simulink model "TITAN_20160720_lec"  (R2016a)
settings: Solver=FixedStepDiscrete  SolverMode=SingleTasking  StartTime=0.0  StopTime=inf  FixedStep=SampleTime  RelTol=1e-3
values from neighbouring files (symbols this model uses):
  LegSampleTime = 0.30    (= 0.3)    [TitanAnalysis_20160720.m]
  SampleTime = 0.05    [TitanAnalysis_20160720.m]
  StepSize = SupportLegStep + IdlingLegStep    [TrajBreakup.m]
undefined symbols (not defined in the file or in its folder): LegTheta
libraries: arduinolib x52, simulink x26, dspswit3 x1
(part 1 of 2)
settings Model: SimulationMode=external  ExtModeTrigDuration=2  Creator=隆  LastModifiedBy=Deckadance
settings DataIOCC: LimitDataPoints=on  SaveFormat=Array
settings OptimizationCC: OptimizeModelRefInitCode=on  LifeSpan=Inf  MaxStackSize=64
settings DebuggingCC: UnderspecifiedInitializationDetection=Classic  MergeDetectMultiDrivingBlocksExec=none  AllowSymbolicDim=off
settings HardwareCC: ProdBitPerInt=16  ProdBitPerPointer=16  ProdLargestAtomicFloat=None  ProdWordSize=8  ProdHWDeviceType=Atmel->AVR  UseEmbeddedCoderFeatures=off  UseSimulinkCoderFeatures=off
settings ModelReferenceCC: PropagateSignalLabelsOutOfModel=off
settings RTWCC: SystemTargetFile=ert.tlc  HardwareBoard=Arduino Mega 2560  TemplateMakefile=ert_default_tmf  RTWVerbose=off  Toolchain=Arduino AVR v1.6.1  BuildConfiguration=Faster Runs
settings CodeAppCC: IgnoreCustomStorageClasses=off
settings ERTTargetCC: SupportContinuousTime=on  SupportNonInlinedSFcns=on  SupportVariableSizeSignals=on  ConvertIfToSwitch=off  SuppressUnreachableDefaultCases=off
settings ConfigComp: CovModelRefEnable=Off

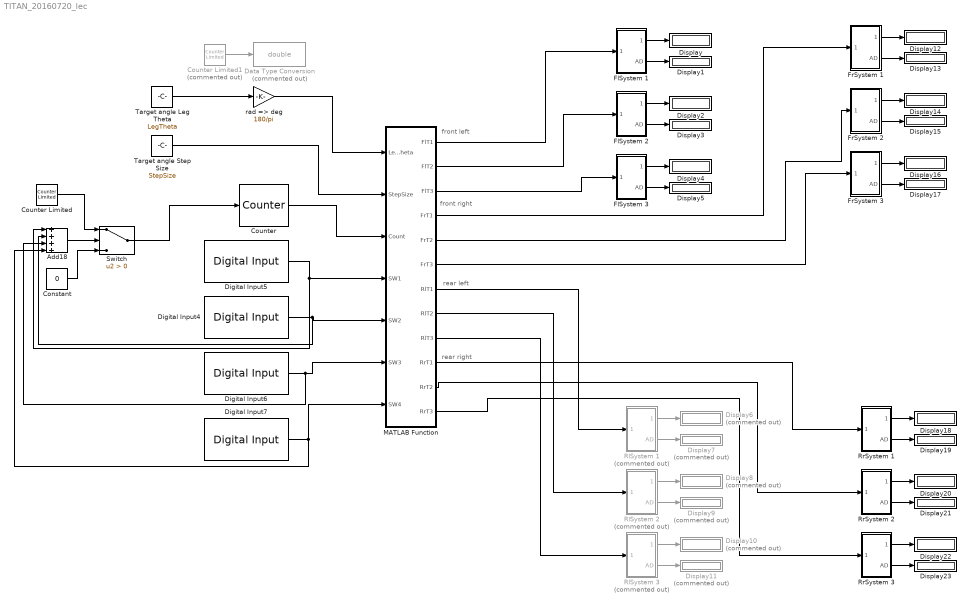
== system TITAN_20160720_lec ==
  note: rear right
  note: rear left
  note: front right
  note: front left
  Add18 : Sum  Inputs=++++
  Constant : Constant  Value=0
  Counter : dspswit3/Counter  Direction=Up  CountEvent=Either edge  CounterSize=User defined  MaxCount=StepSize-1  InitialCount=0  Output=Count  HitValue=32  ResetInput=off  SamplesPerFrame=1  Ts=1  CntDtype=double  HitDtype=Logical
  Counter Limited : simulink/Sources/Counter Limited  uplimit=1  tsamp=LegSampleTime
  Counter Limited1 : simulink/Sources/Counter Limited  Commented=on  uplimit=StepSize-1  tsamp=LegSampleTime
  Data Type Conversion : DataTypeConversion  Commented=on  OutDataTypeStr=double
  Digital Input4 : arduinolib/Digital Input  pinNumber=50  sampleTime=SampleTime  blockPlatform=arduino
  Digital Input5 : arduinolib/Digital Input  pinNumber=51  sampleTime=SampleTime  blockPlatform=arduino
  Digital Input6 : arduinolib/Digital Input  pinNumber=53  sampleTime=SampleTime  blockPlatform=arduino
  Digital Input7 : arduinolib/Digital Input  pinNumber=52  sampleTime=SampleTime  blockPlatform=arduino
  Display{,1..5,12..23} (18 alike) : Display
  Display{6..11} (6 alike) : Display  Commented=on
  FlSystem 1 : Subsystem
  FlSystem 2 : Subsystem
  FlSystem 3 : Subsystem
  FrSystem 1 : Subsystem
  FrSystem 2 : Subsystem
  FrSystem 3 : Subsystem
  MATLAB Function : MATLAB Function  TreatAsAtomicUnit=on
  RlSystem 1 : Subsystem  Commented=on
  RlSystem 2 : Subsystem  Commented=on
  RlSystem 3 : Subsystem  Commented=on
  RrSystem 1 : Subsystem
  RrSystem 2 : Subsystem
  RrSystem 3 : Subsystem
  Switch : Switch  Criteria=u2 > Threshold
  Target angle Leg Theta : Constant  Value=LegTheta  SampleTime=SampleTime
  Target angle Step Size : Constant  Value=StepSize  SampleTime=SampleTime
  rad => deg : Gain  Gain=180/pi
  wires:
  FlSystem 1/1(Angle) -> Display/1
  FlSystem 1/2(AD) -> Display1/1
  FlSystem 2/1(Angle) -> Display2/1
  FlSystem 2/2(AD) -> Display3/1
  FlSystem 3/1(Angle) -> Display4/1
  FlSystem 3/2(AD) -> Display5/1
  RlSystem 1/1(Angle) -> Display6/1
  RlSystem 1/2(AD) -> Display7/1
  RlSystem 2/1(Angle) -> Display8/1
  RlSystem 2/2(AD) -> Display9/1
  RlSystem 3/1(Angle) -> Display10/1
  RlSystem 3/2(AD) -> Display11/1
  FrSystem 1/1(Angle) -> Display12/1
  FrSystem 1/2(AD) -> Display13/1
  FrSystem 2/1(Angle) -> Display14/1
  FrSystem 2/2(AD) -> Display15/1
  FrSystem 3/1(Angle) -> Display16/1
  FrSystem 3/2(AD) -> Display17/1
  RrSystem 1/1(Angle) -> Display18/1
  RrSystem 1/2(AD) -> Display19/1
  RrSystem 2/1(Angle) -> Display20/1
  RrSystem 2/2(AD) -> Display21/1
  RrSystem 3/1(Angle) -> Display22/1
  RrSystem 3/2(AD) -> Display23/1
  MATLAB Function/4(FrT1) -> FrSystem 1/1(In1)
  Counter Limited1/1 -> Data Type Conversion/1
  Target angle Leg Theta/1 -> rad => deg/1
  MATLAB Function/5(FrT2) -> FrSystem 2/1(In1)
  MATLAB Function/6(FrT3) -> FrSystem 3/1(In1)
  MATLAB Function/3(FlT3) -> FlSystem 3/1(In1)
  MATLAB Function/2(FlT2) -> FlSystem 2/1(In1)
  MATLAB Function/1(FlT1) -> FlSystem 1/1(In1)
  MATLAB Function/7(RlT1) -> RlSystem 1/1(In1)
  MATLAB Function/8(RlT2) -> RlSystem 2/1(In1)
  MATLAB Function/9(RlT3) -> RlSystem 3/1(In1)
  MATLAB Function/10(RrT1) -> RrSystem 1/1(In1)
  MATLAB Function/11(RrT2) -> RrSystem 2/1(In1)
  MATLAB Function/12(RrT3) -> RrSystem 3/1(In1)
  Digital Input5/1 -> MATLAB Function/4(SW1), Add18/1
  Digital Input4/1 -> Add18/2, MATLAB Function/5(SW2)
  Counter/1 -> MATLAB Function/3(Count)
  rad => deg/1 -> MATLAB Function/1(LegTheta)
  Digital Input7/1 -> MATLAB Function/7(SW4), Add18/4
  Constant/1 -> Switch/3
  Add18/1 -> Switch/2
  Digital Input6/1 -> MATLAB Function/6(SW3), Add18/3
  Target angle Step Size/1 -> MATLAB Function/2(StepSize)
  Switch/1 -> Counter/1
  Counter Limited/1 -> Switch/1

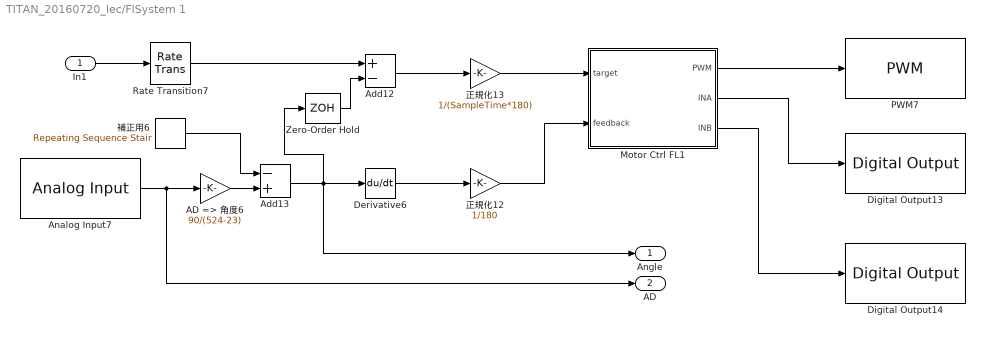
== system TITAN_20160720_lec/FlSystem 1 ==
  In1 : Inport
  AD => 角度6 : Gain  Gain=90/(524-23)
  Add12 : Sum  Inputs=+-
  Add13 : Sum  Inputs=-+
  Analog Input7 : arduinolib/Analog Input  pinNumber=0  sampleTime=SampleTime  blockPlatform=arduino
  Derivative6 : Derivative
  Digital Output13 : arduinolib/Digital Output  pinNumber=34  blockPlatform=arduino
  Digital Output14 : arduinolib/Digital Output  pinNumber=36  blockPlatform=arduino
  Motor Ctrl FL1 : Subsystem
  PWM7 : arduinolib/PWM  pinNumber=8  blockPlatform=arduino
  Rate Transition7 : RateTransition  OutPortSampleTime=SampleTime
  Zero-Order Hold : ZeroOrderHold  SampleTime=LegSampleTime
  正規化12 : Gain  Gain=1/180
  正規化13 : Gain  Gain=1/(SampleTime*180)
  補正用6 : simulink/Sources/Repeating Sequence Stair  OutValues=120.2  tsamp=SampleTime  OutMin=[]  OutMax=[]  OutDataTypeStr=double  OutputDataTypeScalingMode=double  OutDataType=fixdt(0,8)  ConRadixGroup=Best Precision: Vector-wise  OutScaling=2^-12
  Angle : Outport
  AD : Outport  Port=2
  wires:
  Derivative6/1 -> 正規化12/1
  Add13/1 -> Zero-Order Hold/1, Angle/1, Derivative6/1
  Motor Ctrl FL1/2(INA) -> Digital Output13/1
  Motor Ctrl FL1/3(INB) -> Digital Output14/1
  正規化12/1 -> Motor Ctrl FL1/2(feedback)
  Analog Input7/1 -> AD/1, AD => 角度6/1
  Motor Ctrl FL1/1(PWM) -> PWM7/1
  Rate Transition7/1 -> Add12/1
  正規化13/1 -> Motor Ctrl FL1/1(target)
  Add12/1 -> 正規化13/1
  AD => 角度6/1 -> Add13/2
  補正用6/1 -> Add13/1
  In1/1 -> Rate Transition7/1
  Zero-Order Hold/1 -> Add12/2

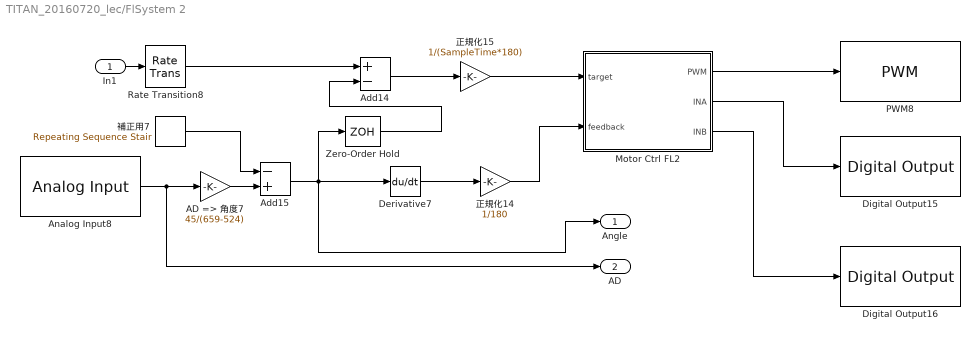
== system TITAN_20160720_lec/FlSystem 2 ==
  In1 : Inport
  AD => 角度7 : Gain  Gain=45/(659-524)
  Add14 : Sum  Inputs=+-
  Add15 : Sum  Inputs=-+
  Analog Input8 : arduinolib/Analog Input  pinNumber=1  sampleTime=SampleTime  blockPlatform=arduino
  Derivative7 : Derivative
  Digital Output15 : arduinolib/Digital Output  pinNumber=35  blockPlatform=arduino
  Digital Output16 : arduinolib/Digital Output  pinNumber=37  blockPlatform=arduino
  Motor Ctrl FL2 : Subsystem
  PWM8 : arduinolib/PWM  pinNumber=9  blockPlatform=arduino
  Rate Transition8 : RateTransition  OutPortSampleTime=SampleTime
  Zero-Order Hold : ZeroOrderHold  SampleTime=LegSampleTime
  正規化14 : Gain  Gain=1/180
  正規化15 : Gain  Gain=1/(SampleTime*180)
  補正用7 : simulink/Sources/Repeating Sequence Stair  OutValues=180  tsamp=SampleTime  OutMin=[]  OutMax=[]  OutDataTypeStr=double  OutputDataTypeScalingMode=double  OutDataType=fixdt(0,8)  ConRadixGroup=Best Precision: Vector-wise  OutScaling=2^-12
  Angle : Outport
  AD : Outport  Port=2
  wires:
  In1/1 -> Rate Transition8/1
  Derivative7/1 -> 正規化14/1
  Add15/1 -> Zero-Order Hold/1, Angle/1, Derivative7/1
  Motor Ctrl FL2/2(INA) -> Digital Output15/1
  Motor Ctrl FL2/3(INB) -> Digital Output16/1
  正規化14/1 -> Motor Ctrl FL2/2(feedback)
  Analog Input8/1 -> AD/1, AD => 角度7/1
  Motor Ctrl FL2/1(PWM) -> PWM8/1
  Rate Transition8/1 -> Add14/1
  正規化15/1 -> Motor Ctrl FL2/1(target)
  Add14/1 -> 正規化15/1
  AD => 角度7/1 -> Add15/2
  補正用7/1 -> Add15/1
  Zero-Order Hold/1 -> Add14/2

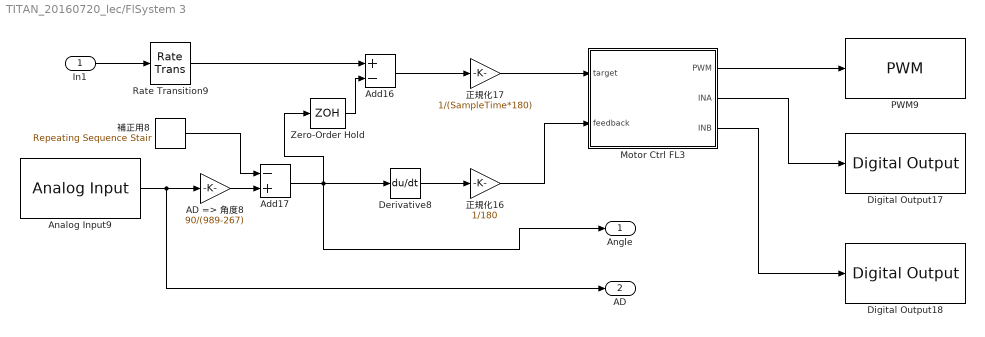
== system TITAN_20160720_lec/FlSystem 3 ==
  In1 : Inport
  AD => 角度8 : Gain  Gain=90/(989-267)
  Add16 : Sum  Inputs=+-
  Add17 : Sum  Inputs=-+
  Analog Input9 : arduinolib/Analog Input  pinNumber=2  sampleTime=SampleTime  blockPlatform=arduino
  Derivative8 : Derivative
  Digital Output17 : arduinolib/Digital Output  pinNumber=41  blockPlatform=arduino
  Digital Output18 : arduinolib/Digital Output  pinNumber=39  blockPlatform=arduino
  Motor Ctrl FL3 : Subsystem
  PWM9 : arduinolib/PWM  pinNumber=11  blockPlatform=arduino
  Rate Transition9 : RateTransition  OutPortSampleTime=SampleTime
  Zero-Order Hold : ZeroOrderHold  SampleTime=LegSampleTime
  正規化16 : Gain  Gain=1/180
  正規化17 : Gain  Gain=1/(SampleTime*180)
  補正用8 : simulink/Sources/Repeating Sequence Stair  OutValues=33.28+90  tsamp=SampleTime  OutMin=[]  OutMax=[]  OutDataTypeStr=double  OutputDataTypeScalingMode=double  OutDataType=fixdt(0,8)  ConRadixGroup=Best Precision: Vector-wise  OutScaling=2^-12
  Angle : Outport
  AD : Outport  Port=2
  wires:
  Derivative8/1 -> 正規化16/1
  Add17/1 -> Zero-Order Hold/1, Angle/1, Derivative8/1
  Motor Ctrl FL3/2(INA) -> Digital Output17/1
  Motor Ctrl FL3/3(INB) -> Digital Output18/1
  正規化16/1 -> Motor Ctrl FL3/2(feedback)
  Analog Input9/1 -> AD/1, AD => 角度8/1
  Motor Ctrl FL3/1(PWM) -> PWM9/1
  Rate Transition9/1 -> Add16/1
  正規化17/1 -> Motor Ctrl FL3/1(target)
  Add16/1 -> 正規化17/1
  AD => 角度8/1 -> Add17/2
  補正用8/1 -> Add17/1
  In1/1 -> Rate Transition9/1
  Zero-Order Hold/1 -> Add16/2

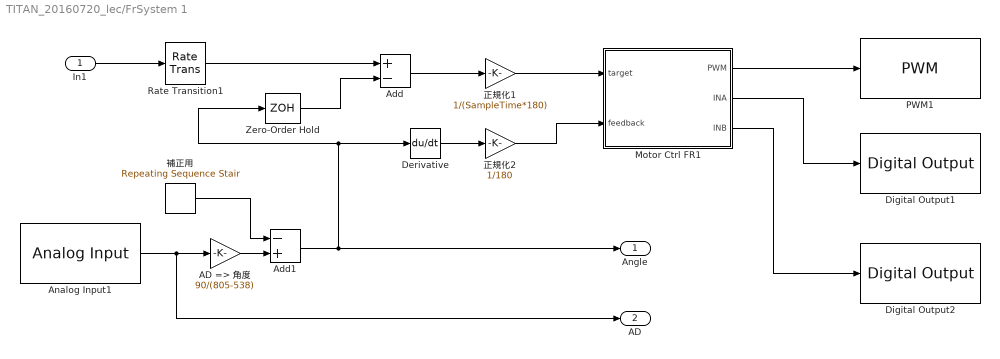
== system TITAN_20160720_lec/FrSystem 1 ==
  In1 : Inport
  AD => 角度 : Gain  Gain=90/(805-538)
  Add : Sum  Inputs=+-
  Add1 : Sum  Inputs=-+
  Analog Input1 : arduinolib/Analog Input  pinNumber=3  sampleTime=SampleTime  blockPlatform=arduino
  Derivative : Derivative
  Digital Output1 : arduinolib/Digital Output  pinNumber=42  blockPlatform=arduino
  Digital Output2 : arduinolib/Digital Output  pinNumber=44  blockPlatform=arduino
  Motor Ctrl FR1 : Subsystem
  PWM1 : arduinolib/PWM  pinNumber=12  blockPlatform=arduino
  Rate Transition1 : RateTransition  OutPortSampleTime=SampleTime
  Zero-Order Hold : ZeroOrderHold  SampleTime=LegSampleTime
  正規化1 : Gain  Gain=1/(SampleTime*180)
  正規化2 : Gain  Gain=1/180
  補正用 : simulink/Sources/Repeating Sequence Stair  OutValues=180  tsamp=SampleTime  OutMin=[]  OutMax=[]  OutDataTypeStr=double  OutputDataTypeScalingMode=double  OutDataType=fixdt(0,8)  ConRadixGroup=Best Precision: Vector-wise  OutScaling=2^-12
  Angle : Outport
  AD : Outport  Port=2
  wires:
  In1/1 -> Rate Transition1/1
  Motor Ctrl FR1/2(INA) -> Digital Output1/1
  Motor Ctrl FR1/3(INB) -> Digital Output2/1
  Derivative/1 -> 正規化2/1
  Analog Input1/1 -> AD/1, AD => 角度/1
  Motor Ctrl FR1/1(PWM) -> PWM1/1
  Rate Transition1/1 -> Add/1
  AD => 角度/1 -> Add1/2
  Add/1 -> 正規化1/1
  補正用/1 -> Add1/1
  正規化1/1 -> Motor Ctrl FR1/1(target)
  正規化2/1 -> Motor Ctrl FR1/2(feedback)
  Add1/1 -> Derivative/1, Zero-Order Hold/1, Angle/1
  Zero-Order Hold/1 -> Add/2

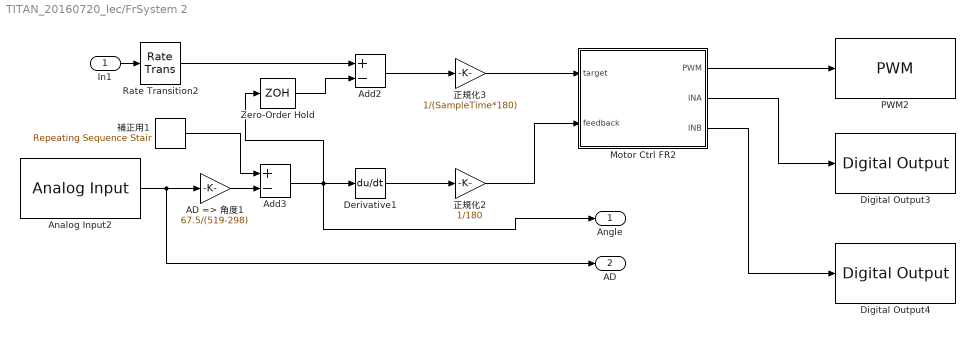
== system TITAN_20160720_lec/FrSystem 2 ==
  In1 : Inport
  AD => 角度1 : Gain  Gain=67.5/(519-298)
  Add2 : Sum  Inputs=+-
  Add3 : Sum  Inputs=+-
  Analog Input2 : arduinolib/Analog Input  pinNumber=4  sampleTime=SampleTime  blockPlatform=arduino
  Derivative1 : Derivative
  Digital Output3 : arduinolib/Digital Output  pinNumber=45  blockPlatform=arduino
  Digital Output4 : arduinolib/Digital Output  pinNumber=43  blockPlatform=arduino
  Motor Ctrl FR2 : Subsystem
  PWM2 : arduinolib/PWM  pinNumber=13  blockPlatform=arduino
  Rate Transition2 : RateTransition  OutPortSampleTime=SampleTime
  Zero-Order Hold : ZeroOrderHold  SampleTime=LegSampleTime
  正規化2 : Gain  Gain=1/180
  正規化3 : Gain  Gain=1/(SampleTime*180)
  補正用1 : simulink/Sources/Repeating Sequence Stair  OutValues=158.5  tsamp=SampleTime  OutMin=[]  OutMax=[]  OutDataTypeStr=double  OutputDataTypeScalingMode=double  OutDataType=fixdt(0,8)  ConRadixGroup=Best Precision: Vector-wise  OutScaling=2^-12
  Angle : Outport
  AD : Outport  Port=2
  wires:
  In1/1 -> Rate Transition2/1
  Derivative1/1 -> 正規化2/1
  Add3/1 -> Angle/1, Zero-Order Hold/1, Derivative1/1
  Motor Ctrl FR2/2(INA) -> Digital Output3/1
  Motor Ctrl FR2/3(INB) -> Digital Output4/1
  正規化2/1 -> Motor Ctrl FR2/2(feedback)
  Analog Input2/1 -> AD/1, AD => 角度1/1
  Motor Ctrl FR2/1(PWM) -> PWM2/1
  正規化3/1 -> Motor Ctrl FR2/1(target)
  Rate Transition2/1 -> Add2/1
  Add2/1 -> 正規化3/1
  AD => 角度1/1 -> Add3/2
  補正用1/1 -> Add3/1
  Zero-Order Hold/1 -> Add2/2

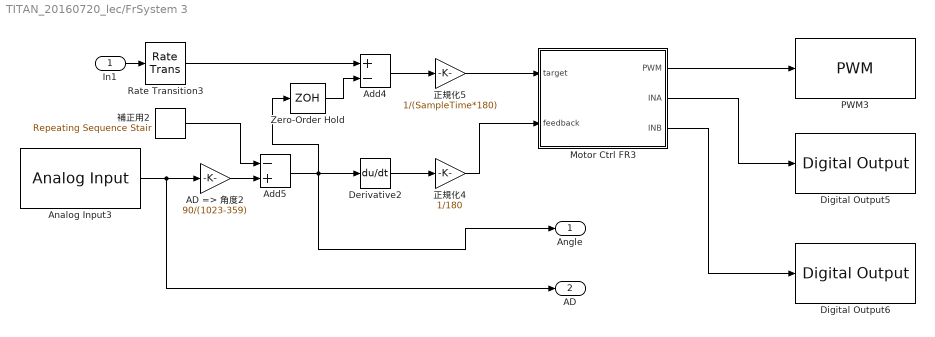
== system TITAN_20160720_lec/FrSystem 3 ==
  In1 : Inport
  AD => 角度2 : Gain  Gain=90/(1023-359)
  Add4 : Sum  Inputs=+-
  Add5 : Sum  Inputs=-+
  Analog Input3 : arduinolib/Analog Input  pinNumber=5  sampleTime=SampleTime  blockPlatform=arduino
  Derivative2 : Derivative
  Digital Output5 : arduinolib/Digital Output  pinNumber=38  blockPlatform=arduino
  Digital Output6 : arduinolib/Digital Output  pinNumber=40  blockPlatform=arduino
  Motor Ctrl FR3 : Subsystem
  PWM3 : arduinolib/PWM  pinNumber=10  blockPlatform=arduino
  Rate Transition3 : RateTransition  OutPortSampleTime=SampleTime
  Zero-Order Hold : ZeroOrderHold  SampleTime=LegSampleTime
  正規化4 : Gain  Gain=1/180
  正規化5 : Gain  Gain=1/(SampleTime*180)
  補正用2 : simulink/Sources/Repeating Sequence Stair  OutValues=47.3+90  tsamp=SampleTime  OutMin=[]  OutMax=[]  OutDataTypeStr=double  OutputDataTypeScalingMode=double  OutDataType=fixdt(0,8)  ConRadixGroup=Best Precision: Vector-wise  OutScaling=2^-12
  Angle : Outport
  AD : Outport  Port=2
  wires:
  In1/1 -> Rate Transition3/1
  Derivative2/1 -> 正規化4/1
  Add5/1 -> Zero-Order Hold/1, Angle/1, Derivative2/1
  Motor Ctrl FR3/2(INA) -> Digital Output5/1
  Motor Ctrl FR3/3(INB) -> Digital Output6/1
  正規化4/1 -> Motor Ctrl FR3/2(feedback)
  Analog Input3/1 -> AD/1, AD => 角度2/1
  Motor Ctrl FR3/1(PWM) -> PWM3/1
  Rate Transition3/1 -> Add4/1
  Add4/1 -> 正規化5/1
  AD => 角度2/1 -> Add5/2
  補正用2/1 -> Add5/1
  正規化5/1 -> Motor Ctrl FR3/1(target)
  Zero-Order Hold/1 -> Add4/2

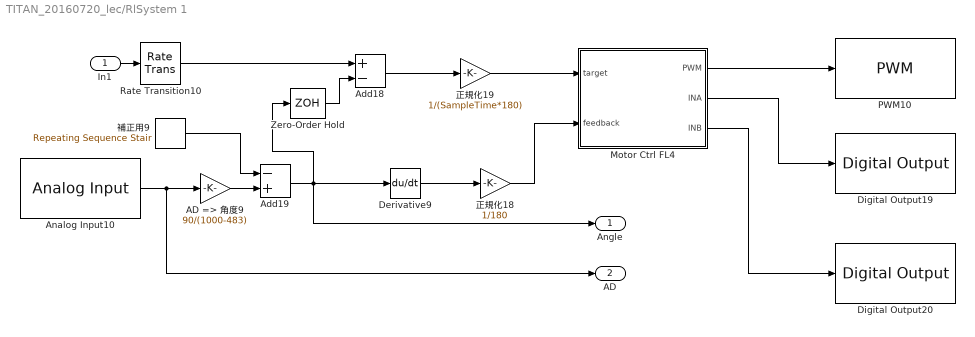
== system TITAN_20160720_lec/RlSystem 1 ==
  In1 : Inport
  AD => 角度9 : Gain  Gain=90/(1000-483)
  Add18 : Sum  Inputs=+-
  Add19 : Sum  Inputs=-+
  Analog Input10 : arduinolib/Analog Input  pinNumber=9  sampleTime=SampleTime  blockPlatform=arduino
  Derivative9 : Derivative
  Digital Output19 : arduinolib/Digital Output  pinNumber=30  blockPlatform=arduino
  Digital Output20 : arduinolib/Digital Output  pinNumber=32  blockPlatform=arduino
  Motor Ctrl FL4 : Subsystem
  PWM10 : arduinolib/PWM  pinNumber=6  blockPlatform=arduino
  Rate Transition10 : RateTransition  OutPortSampleTime=SampleTime
  Zero-Order Hold : ZeroOrderHold  SampleTime=LegSampleTime
  正規化18 : Gain  Gain=1/180
  正規化19 : Gain  Gain=1/(SampleTime*180)
  補正用9 : simulink/Sources/Repeating Sequence Stair  OutValues=83.38  tsamp=SampleTime  OutMin=[]  OutMax=[]  OutDataTypeStr=double  OutputDataTypeScalingMode=double  OutDataType=fixdt(0,8)  ConRadixGroup=Best Precision: Vector-wise  OutScaling=2^-12
  Angle : Outport
  AD : Outport  Port=2
  wires:
  In1/1 -> Rate Transition10/1
  Derivative9/1 -> 正規化18/1
  Add19/1 -> Zero-Order Hold/1, Angle/1, Derivative9/1
  Motor Ctrl FL4/2(INA) -> Digital Output19/1
  Motor Ctrl FL4/3(INB) -> Digital Output20/1
  正規化18/1 -> Motor Ctrl FL4/2(feedback)
  Analog Input10/1 -> AD/1, AD => 角度9/1
  Motor Ctrl FL4/1(PWM) -> PWM10/1
  Rate Transition10/1 -> Add18/1
  正規化19/1 -> Motor Ctrl FL4/1(target)
  Add18/1 -> 正規化19/1
  AD => 角度9/1 -> Add19/2
  補正用9/1 -> Add19/1
  Zero-Order Hold/1 -> Add18/2

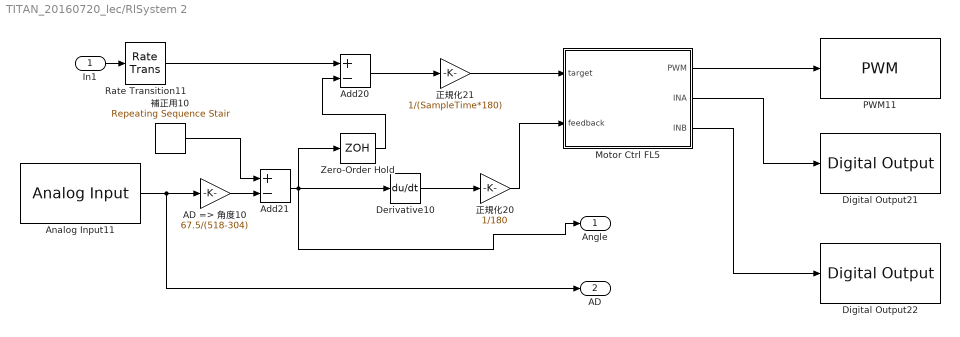
== system TITAN_20160720_lec/RlSystem 2 ==
  In1 : Inport
  AD => 角度10 : Gain  Gain=67.5/(518-304)
  Add20 : Sum  Inputs=+-
  Add21 : Sum  Inputs=+-
  Analog Input11 : arduinolib/Analog Input  pinNumber=10  sampleTime=SampleTime  blockPlatform=arduino
  Derivative10 : Derivative
  Digital Output21 : arduinolib/Digital Output  pinNumber=33  blockPlatform=arduino
  Digital Output22 : arduinolib/Digital Output  pinNumber=31  blockPlatform=arduino
  Motor Ctrl FL5 : Subsystem
  PWM11 : arduinolib/PWM  pinNumber=7  blockPlatform=arduino
  Rate Transition11 : RateTransition  OutPortSampleTime=SampleTime
  Zero-Order Hold : ZeroOrderHold  SampleTime=LegSampleTime
  正規化20 : Gain  Gain=1/180
  正規化21 : Gain  Gain=1/(SampleTime*180)
  補正用10 : simulink/Sources/Repeating Sequence Stair  OutValues=161.5  tsamp=SampleTime  OutMin=[]  OutMax=[]  OutDataTypeStr=double  OutputDataTypeScalingMode=double  OutDataType=fixdt(0,8)  ConRadixGroup=Best Precision: Vector-wise  OutScaling=2^-12
  Angle : Outport
  AD : Outport  Port=2
  wires:
  In1/1 -> Rate Transition11/1
  Derivative10/1 -> 正規化20/1
  Add21/1 -> Zero-Order Hold/1, Angle/1, Derivative10/1
  Motor Ctrl FL5/2(INA) -> Digital Output21/1
  Motor Ctrl FL5/3(INB) -> Digital Output22/1
  正規化20/1 -> Motor Ctrl FL5/2(feedback)
  Analog Input11/1 -> AD/1, AD => 角度10/1
  Motor Ctrl FL5/1(PWM) -> PWM11/1
  Rate Transition11/1 -> Add20/1
  正規化21/1 -> Motor Ctrl FL5/1(target)
  Add20/1 -> 正規化21/1
  AD => 角度10/1 -> Add21/2
  補正用10/1 -> Add21/1
  Zero-Order Hold/1 -> Add20/2

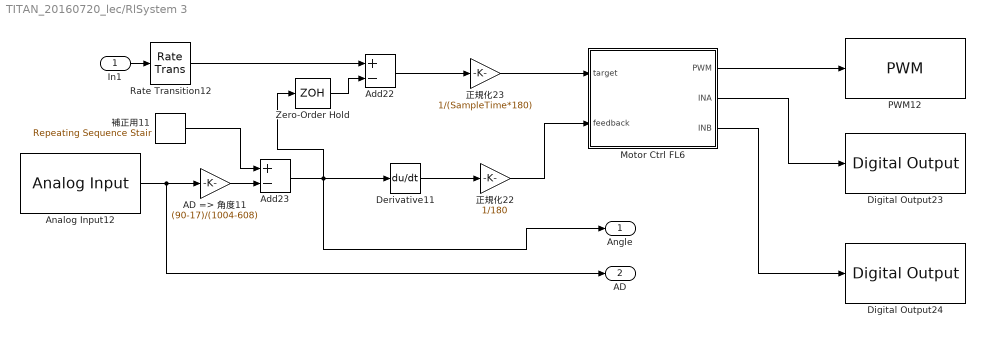
== system TITAN_20160720_lec/RlSystem 3 ==
  In1 : Inport
  AD => 角度11 : Gain  Gain=(90-17)/(1004-608)
  Add22 : Sum  Inputs=+-
  Add23 : Sum  Inputs=+-
  Analog Input12 : arduinolib/Analog Input  pinNumber=11  sampleTime=SampleTime  blockPlatform=arduino
  Derivative11 : Derivative
  Digital Output23 : arduinolib/Digital Output  pinNumber=26  blockPlatform=arduino
  Digital Output24 : arduinolib/Digital Output  pinNumber=28  blockPlatform=arduino
  Motor Ctrl FL6 : Subsystem
  PWM12 : arduinolib/PWM  pinNumber=4  blockPlatform=arduino
  Rate Transition12 : RateTransition  OutPortSampleTime=SampleTime
  Zero-Order Hold : ZeroOrderHold  SampleTime=LegSampleTime
  正規化22 : Gain  Gain=1/180
  正規化23 : Gain  Gain=1/(SampleTime*180)
  補正用11 : simulink/Sources/Repeating Sequence Stair  OutValues=110-90  tsamp=SampleTime  OutMin=[]  OutMax=[]  OutDataTypeStr=double  OutputDataTypeScalingMode=double  OutDataType=fixdt(0,8)  ConRadixGroup=Best Precision: Vector-wise  OutScaling=2^-12
  Angle : Outport
  AD : Outport  Port=2
  wires:
  Derivative11/1 -> 正規化22/1
  Motor Ctrl FL6/2(INA) -> Digital Output23/1
  Motor Ctrl FL6/3(INB) -> Digital Output24/1
  正規化22/1 -> Motor Ctrl FL6/2(feedback)
  Analog Input12/1 -> AD/1, AD => 角度11/1
  Motor Ctrl FL6/1(PWM) -> PWM12/1
  Rate Transition12/1 -> Add22/1
  正規化23/1 -> Motor Ctrl FL6/1(target)
  Add22/1 -> 正規化23/1
  AD => 角度11/1 -> Add23/2
  補正用11/1 -> Add23/1
  In1/1 -> Rate Transition12/1
  Zero-Order Hold/1 -> Add22/2
  Add23/1 -> Zero-Order Hold/1, Angle/1, Derivative11/1

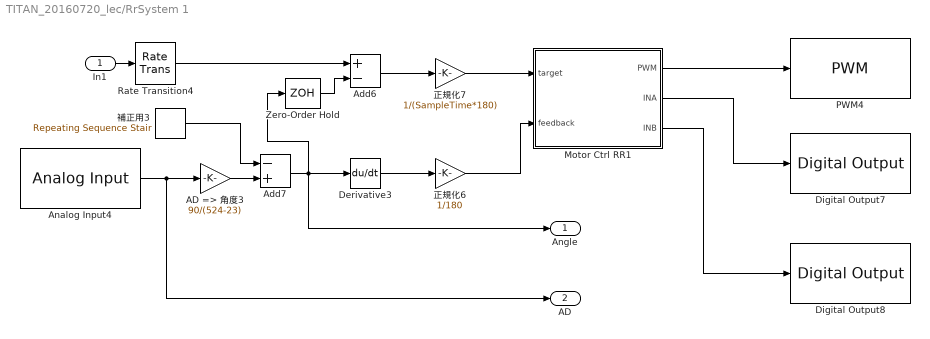
== system TITAN_20160720_lec/RrSystem 1 ==
  In1 : Inport
  AD => 角度3 : Gain  Gain=90/(524-23)
  Add6 : Sum  Inputs=+-
  Add7 : Sum  Inputs=-+
  Analog Input4 : arduinolib/Analog Input  pinNumber=6  sampleTime=SampleTime  blockPlatform=arduino
  Derivative3 : Derivative
  Digital Output7 : arduinolib/Digital Output  pinNumber=22  blockPlatform=arduino
  Digital Output8 : arduinolib/Digital Output  pinNumber=24  blockPlatform=arduino
  Motor Ctrl RR1 : Subsystem
  PWM4 : arduinolib/PWM  pinNumber=2  blockPlatform=arduino
  Rate Transition4 : RateTransition  OutPortSampleTime=SampleTime
  Zero-Order Hold : ZeroOrderHold  SampleTime=LegSampleTime
  正規化6 : Gain  Gain=1/180
  正規化7 : Gain  Gain=1/(SampleTime*180)
  補正用3 : simulink/Sources/Repeating Sequence Stair  OutValues=93.77  tsamp=SampleTime  OutMin=[]  OutMax=[]  OutDataTypeStr=double  OutputDataTypeScalingMode=double  OutDataType=fixdt(0,8)  ConRadixGroup=Best Precision: Vector-wise  OutScaling=2^-12
  Angle : Outport
  AD : Outport  Port=2
  wires:
  In1/1 -> Rate Transition4/1
  Derivative3/1 -> 正規化6/1
  Add7/1 -> Zero-Order Hold/1, Angle/1, Derivative3/1
  Motor Ctrl RR1/2(INA) -> Digital Output7/1
  Motor Ctrl RR1/3(INB) -> Digital Output8/1
  正規化6/1 -> Motor Ctrl RR1/2(feedback)
  Analog Input4/1 -> AD/1, AD => 角度3/1
  Motor Ctrl RR1/1(PWM) -> PWM4/1
  Rate Transition4/1 -> Add6/1
  Add6/1 -> 正規化7/1
  正規化7/1 -> Motor Ctrl RR1/1(target)
  補正用3/1 -> Add7/1
  AD => 角度3/1 -> Add7/2
  Zero-Order Hold/1 -> Add6/2

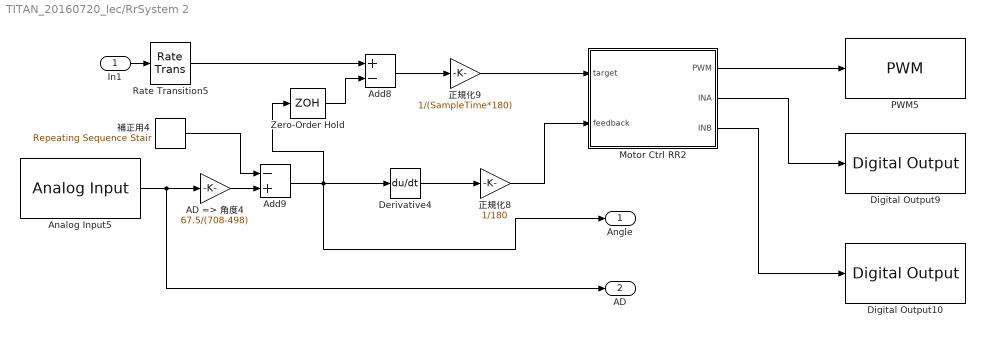
== system TITAN_20160720_lec/RrSystem 2 ==
  In1 : Inport
  AD => 角度4 : Gain  Gain=67.5/(708-498)
  Add8 : Sum  Inputs=+-
  Add9 : Sum  Inputs=-+
  Analog Input5 : arduinolib/Analog Input  pinNumber=7  sampleTime=SampleTime  blockPlatform=arduino
  Derivative4 : Derivative
  Digital Output10 : arduinolib/Digital Output  pinNumber=25  blockPlatform=arduino
  Digital Output9 : arduinolib/Digital Output  pinNumber=23  blockPlatform=arduino
  Motor Ctrl RR2 : Subsystem
  PWM5 : arduinolib/PWM  pinNumber=3  blockPlatform=arduino
  Rate Transition5 : RateTransition  OutPortSampleTime=SampleTime
  Zero-Order Hold : ZeroOrderHold  SampleTime=LegSampleTime
  正規化8 : Gain  Gain=1/180
  正規化9 : Gain  Gain=1/(SampleTime*180)
  補正用4 : simulink/Sources/Repeating Sequence Stair  OutValues=160.7  tsamp=SampleTime  OutMin=[]  OutMax=[]  OutDataTypeStr=double  OutputDataTypeScalingMode=double  OutDataType=fixdt(0,8)  ConRadixGroup=Best Precision: Vector-wise  OutScaling=2^-12
  Angle : Outport
  AD : Outport  Port=2
  wires:
  In1/1 -> Rate Transition5/1
  Derivative4/1 -> 正規化8/1
  Add9/1 -> Zero-Order Hold/1, Angle/1, Derivative4/1
  Motor Ctrl RR2/2(INA) -> Digital Output9/1
  Motor Ctrl RR2/3(INB) -> Digital Output10/1
  正規化8/1 -> Motor Ctrl RR2/2(feedback)
  Analog Input5/1 -> AD/1, AD => 角度4/1
  Motor Ctrl RR2/1(PWM) -> PWM5/1
  Rate Transition5/1 -> Add8/1
  正規化9/1 -> Motor Ctrl RR2/1(target)
  Add8/1 -> 正規化9/1
  AD => 角度4/1 -> Add9/2
  補正用4/1 -> Add9/1
  Zero-Order Hold/1 -> Add8/2

== system TITAN_20160720_lec/RrSystem 3 ==
  In1 : Inport
  AD => 角度5 : Gain  Gain=(134-17)/(1003-21)
  Add10 : Sum  Inputs=+-
  Add11 : Sum  Inputs=+-
  Analog Input6 : arduinolib/Analog Input  pinNumber=8  sampleTime=SampleTime  blockPlatform=arduino
  Derivative5 : Derivative
  Digital Output11 : arduinolib/Digital Output  pinNumber=29  blockPlatform=arduino
  Digital Output12 : arduinolib/Digital Output  pinNumber=27  blockPlatform=arduino
  Motor Ctrl RR3 : Subsystem
  PWM6 : arduinolib/PWM  pinNumber=5  blockPlatform=arduino
  Rate Transition6 : RateTransition  OutPortSampleTime=SampleTime
  Zero-Order Hold : ZeroOrderHold  SampleTime=LegSampleTime
  正規化10 : Gain  Gain=1/180
  正規化11 : Gain  Gain=1/(SampleTime*180)
  補正用5 : simulink/Sources/Repeating Sequence Stair  OutValues=78.06-90  tsamp=SampleTime  OutMin=[]  OutMax=[]  OutDataTypeStr=double  OutputDataTypeScalingMode=double  OutDataType=fixdt(0,8)  ConRadixGroup=Best Precision: Vector-wise  OutScaling=2^-12
  Angle : Outport
  AD : Outport  Port=2
  wires:
  In1/1 -> Rate Transition6/1
  Derivative5/1 -> 正規化10/1
  Add11/1 -> Zero-Order Hold/1, Angle/1, Derivative5/1
  Motor Ctrl RR3/2(INA) -> Digital Output11/1
  Motor Ctrl RR3/3(INB) -> Digital Output12/1
  正規化10/1 -> Motor Ctrl RR3/2(feedback)
  Analog Input6/1 -> AD/1, AD => 角度5/1
  Motor Ctrl RR3/1(PWM) -> PWM6/1
  Rate Transition6/1 -> Add10/1
  Add10/1 -> 正規化11/1
  正規化11/1 -> Motor Ctrl RR3/1(target)
  補正用5/1 -> Add11/1
  AD => 角度5/1 -> Add11/2
  Zero-Order Hold/1 -> Add10/2

== system TITAN_20160720_lec/FlSystem 1/Motor Ctrl FL1 ==
  note: motor driver
  target : Inport
  feedback : Inport  Port=2
  Abs : Abs
  Add : Sum  Inputs=+-
  Discrete PID Controller : simulink/Continuous/PID Controller  Controller=PID  TimeDomain=Discrete-time  SampleTime=SampleTime  IntegratorMethod=Trapezoidal  FilterMethod=Forward Euler  Form=Parallel  UseFilter=on  ControllerParametersSource=internal  P=0.25  I=0  D=0  N=100  InitialConditionSource=internal  InitialConditionForIntegrator=0  InitialConditionForFilter=0  ExternalReset=none  LimitOutput=on  UpperSaturationLimit=1  LowerSaturationLimit=-1  LinearizeAsGain=off  AntiWindupMode=none  Kb=1  TrackingMode=off  Kt=1  PParamMin=[]  PParamMax=[]  IParamMin=[]  IParamMax=[]  DParamMin=[]  DParamMax=[]  NParamMin=[]  NParamMax=[]  KbParamMin=[]  KbParamMax=[]  KtParamMin=[]  KtParamMax=[]  POutMin=[]  POutMax=[]  IOutMin=[]  IOutMax=[]  DOutMin=[]  DOutMax=[]  NOutMin=[]  NOutMax=[]  KbOutMin=[]  KbOutMax=[]  KtOutMin=[]  KtOutMax=[]  IntegratorOutMin=[]  IntegratorOutMax=[]  FilterOutMin=[]  FilterOutMax=[]  SumOutMin=[]  SumOutMax=[]  SumI1OutMin=[]  SumI1OutMax=[]  SumI2OutMin=[]  SumI2OutMax=[]  SumI3OutMin=[]  SumI3OutMax=[]  SumDOutMin=[]  SumDOutMax=[]  SaturationOutMin=[]  SaturationOutMax=[]  IntegratorContinuousStateAttributes=''  IntegratorStateMustResolveToSignalObject=off  IntegratorRTWStateStorageClass=Auto  FilterContinuousStateAttributes=''  FilterStateMustResolveToSignalObject=off  FilterRTWStateStorageClass=Auto  DifferentiatorICPrevScaledInput=0  DifferentiatorOutMin=[]  DifferentiatorOutMax=[]
  Gain : Gain  Gain=255
  Saturation : Saturate  UpperLimit=1  LowerLimit=0
  Saturation1 : Saturate  UpperLimit=1  LowerLimit=0
  Saturation2 : Saturate  UpperLimit=1  LowerLimit=0
  Sign : Signum
  Unary Minus : UnaryMinus
  PWM : Outport
  INA : Outport  Port=2
  INB : Outport  Port=3
  wires:
  feedback/1 -> Add/2
  Abs/1 -> Saturation2/1
  Sign/1 -> Unary Minus/1, Saturation/1
  Discrete PID Controller/1 -> Abs/1, Sign/1
  Saturation/1 -> INA/1
  Saturation1/1 -> INB/1
  Unary Minus/1 -> Saturation1/1
  target/1 -> Add/1
  Saturation2/1 -> Gain/1
  Gain/1 -> PWM/1
  Add/1 -> Discrete PID Controller/1

== system TITAN_20160720_lec/FlSystem 2/Motor Ctrl FL2 ==
  target : Inport
  feedback : Inport  Port=2
  Abs : Abs
  Add : Sum  Inputs=+-
  Discrete PID Controller : simulink/Continuous/PID Controller  Controller=PID  TimeDomain=Discrete-time  SampleTime=SampleTime  IntegratorMethod=Trapezoidal  FilterMethod=Forward Euler  Form=Parallel  UseFilter=on  ControllerParametersSource=internal  P=0.2  I=0  D=0  N=100  InitialConditionSource=internal  InitialConditionForIntegrator=0  InitialConditionForFilter=0  ExternalReset=none  LimitOutput=on  UpperSaturationLimit=1  LowerSaturationLimit=-1  LinearizeAsGain=off  AntiWindupMode=none  Kb=1  TrackingMode=off  Kt=1  PParamMin=[]  PParamMax=[]  IParamMin=[]  IParamMax=[]  DParamMin=[]  DParamMax=[]  NParamMin=[]  NParamMax=[]  KbParamMin=[]  KbParamMax=[]  KtParamMin=[]  KtParamMax=[]  POutMin=[]  POutMax=[]  IOutMin=[]  IOutMax=[]  DOutMin=[]  DOutMax=[]  NOutMin=[]  NOutMax=[]  KbOutMin=[]  KbOutMax=[]  KtOutMin=[]  KtOutMax=[]  IntegratorOutMin=[]  IntegratorOutMax=[]  FilterOutMin=[]  FilterOutMax=[]  SumOutMin=[]  SumOutMax=[]  SumI1OutMin=[]  SumI1OutMax=[]  SumI2OutMin=[]  SumI2OutMax=[]  SumI3OutMin=[]  SumI3OutMax=[]  SumDOutMin=[]  SumDOutMax=[]  SaturationOutMin=[]  SaturationOutMax=[]  IntegratorContinuousStateAttributes=''  IntegratorStateMustResolveToSignalObject=off  IntegratorRTWStateStorageClass=Auto  FilterContinuousStateAttributes=''  FilterStateMustResolveToSignalObject=off  FilterRTWStateStorageClass=Auto  DifferentiatorICPrevScaledInput=0  DifferentiatorOutMin=[]  DifferentiatorOutMax=[]
  Gain : Gain  Gain=255
  Saturation : Saturate  UpperLimit=1  LowerLimit=0
  Saturation1 : Saturate  UpperLimit=1  LowerLimit=0
  Saturation2 : Saturate  UpperLimit=1  LowerLimit=0
  Sign : Signum
  Unary Minus : UnaryMinus
  PWM : Outport
  INA : Outport  Port=2
  INB : Outport  Port=3
  wires:
  feedback/1 -> Add/2
  Abs/1 -> Saturation2/1
  Sign/1 -> Unary Minus/1, Saturation/1
  Discrete PID Controller/1 -> Abs/1, Sign/1
  Saturation/1 -> INA/1
  Saturation1/1 -> INB/1
  Unary Minus/1 -> Saturation1/1
  target/1 -> Add/1
  Saturation2/1 -> Gain/1
  Gain/1 -> PWM/1
  Add/1 -> Discrete PID Controller/1

== system TITAN_20160720_lec/FlSystem 3/Motor Ctrl FL3 ==
  target : Inport
  feedback : Inport  Port=2
  Abs : Abs
  Add : Sum  Inputs=+-
  Discrete PID Controller : simulink/Continuous/PID Controller  Controller=PID  TimeDomain=Discrete-time  SampleTime=SampleTime  IntegratorMethod=Trapezoidal  FilterMethod=Forward Euler  Form=Parallel  UseFilter=on  ControllerParametersSource=internal  P=0.2  I=0  D=0  N=100  InitialConditionSource=internal  InitialConditionForIntegrator=0  InitialConditionForFilter=0  ExternalReset=none  LimitOutput=on  UpperSaturationLimit=1  LowerSaturationLimit=-1  LinearizeAsGain=off  AntiWindupMode=none  Kb=1  TrackingMode=off  Kt=1  PParamMin=[]  PParamMax=[]  IParamMin=[]  IParamMax=[]  DParamMin=[]  DParamMax=[]  NParamMin=[]  NParamMax=[]  KbParamMin=[]  KbParamMax=[]  KtParamMin=[]  KtParamMax=[]  POutMin=[]  POutMax=[]  IOutMin=[]  IOutMax=[]  DOutMin=[]  DOutMax=[]  NOutMin=[]  NOutMax=[]  KbOutMin=[]  KbOutMax=[]  KtOutMin=[]  KtOutMax=[]  IntegratorOutMin=[]  IntegratorOutMax=[]  FilterOutMin=[]  FilterOutMax=[]  SumOutMin=[]  SumOutMax=[]  SumI1OutMin=[]  SumI1OutMax=[]  SumI2OutMin=[]  SumI2OutMax=[]  SumI3OutMin=[]  SumI3OutMax=[]  SumDOutMin=[]  SumDOutMax=[]  SaturationOutMin=[]  SaturationOutMax=[]  IntegratorContinuousStateAttributes=''  IntegratorStateMustResolveToSignalObject=off  IntegratorRTWStateStorageClass=Auto  FilterContinuousStateAttributes=''  FilterStateMustResolveToSignalObject=off  FilterRTWStateStorageClass=Auto  DifferentiatorICPrevScaledInput=0  DifferentiatorOutMin=[]  DifferentiatorOutMax=[]
  Gain : Gain  Gain=255
  Saturation : Saturate  UpperLimit=1  LowerLimit=0
  Saturation1 : Saturate  UpperLimit=1  LowerLimit=0
  Saturation2 : Saturate  LowerLimit=0
  Sign : Signum
  Unary Minus : UnaryMinus
  PWM : Outport
  INA : Outport  Port=2
  INB : Outport  Port=3
  wires:
  feedback/1 -> Add/2
  Abs/1 -> Saturation2/1
  Sign/1 -> Unary Minus/1, Saturation/1
  Discrete PID Controller/1 -> Abs/1, Sign/1
  Saturation/1 -> INA/1
  Saturation1/1 -> INB/1
  Unary Minus/1 -> Saturation1/1
  target/1 -> Add/1
  Saturation2/1 -> Gain/1
  Gain/1 -> PWM/1
  Add/1 -> Discrete PID Controller/1

== system TITAN_20160720_lec/FrSystem 1/Motor Ctrl FR1 ==
  target : Inport
  feedback : Inport  Port=2
  Abs : Abs
  Add : Sum  Inputs=+-
  Discrete PID Controller : simulink/Continuous/PID Controller  Controller=PID  TimeDomain=Discrete-time  SampleTime=SampleTime  IntegratorMethod=Trapezoidal  FilterMethod=Forward Euler  Form=Parallel  UseFilter=on  ControllerParametersSource=internal  P=0.4  I=0  D=0  N=100  InitialConditionSource=internal  InitialConditionForIntegrator=0  InitialConditionForFilter=0  ExternalReset=none  LimitOutput=on  UpperSaturationLimit=1  LowerSaturationLimit=-1  LinearizeAsGain=off  AntiWindupMode=none  Kb=1  TrackingMode=off  Kt=1  PParamMin=[]  PParamMax=[]  IParamMin=[]  IParamMax=[]  DParamMin=[]  DParamMax=[]  NParamMin=[]  NParamMax=[]  KbParamMin=[]  KbParamMax=[]  KtParamMin=[]  KtParamMax=[]  POutMin=[]  POutMax=[]  IOutMin=[]  IOutMax=[]  DOutMin=[]  DOutMax=[]  NOutMin=[]  NOutMax=[]  KbOutMin=[]  KbOutMax=[]  KtOutMin=[]  KtOutMax=[]  IntegratorOutMin=[]  IntegratorOutMax=[]  FilterOutMin=[]  FilterOutMax=[]  SumOutMin=[]  SumOutMax=[]  SumI1OutMin=[]  SumI1OutMax=[]  SumI2OutMin=[]  SumI2OutMax=[]  SumI3OutMin=[]  SumI3OutMax=[]  SumDOutMin=[]  SumDOutMax=[]  SaturationOutMin=[]  SaturationOutMax=[]  IntegratorContinuousStateAttributes=''  IntegratorStateMustResolveToSignalObject=off  IntegratorRTWStateStorageClass=Auto  FilterContinuousStateAttributes=''  FilterStateMustResolveToSignalObject=off  FilterRTWStateStorageClass=Auto  DifferentiatorICPrevScaledInput=0  DifferentiatorOutMin=[]  DifferentiatorOutMax=[]
  Gain : Gain  Gain=255
  Saturation : Saturate  UpperLimit=1  LowerLimit=0
  Saturation1 : Saturate  UpperLimit=1  LowerLimit=0
  Saturation2 : Saturate  UpperLimit=1  LowerLimit=0
  Sign : Signum
  Unary Minus : UnaryMinus
  PWM : Outport
  INA : Outport  Port=2
  INB : Outport  Port=3
  wires:
  feedback/1 -> Add/2
  Abs/1 -> Saturation2/1
  Sign/1 -> Unary Minus/1, Saturation/1
  Discrete PID Controller/1 -> Abs/1, Sign/1
  Saturation/1 -> INA/1
  Saturation1/1 -> INB/1
  Unary Minus/1 -> Saturation1/1
  target/1 -> Add/1
  Saturation2/1 -> Gain/1
  Gain/1 -> PWM/1
  Add/1 -> Discrete PID Controller/1

== system TITAN_20160720_lec/FrSystem 2/Motor Ctrl FR2 ==
  target : Inport
  feedback : Inport  Port=2
  Abs : Abs
  Add : Sum  Inputs=+-
  Discrete PID Controller : simulink/Continuous/PID Controller  Controller=PID  TimeDomain=Discrete-time  SampleTime=SampleTime  IntegratorMethod=Trapezoidal  FilterMethod=Forward Euler  Form=Parallel  UseFilter=on  ControllerParametersSource=internal  P=0.3  I=0  D=0  N=100  InitialConditionSource=internal  InitialConditionForIntegrator=0  InitialConditionForFilter=0  ExternalReset=none  LimitOutput=on  UpperSaturationLimit=1  LowerSaturationLimit=-1  LinearizeAsGain=off  AntiWindupMode=none  Kb=1  TrackingMode=off  Kt=1  PParamMin=[]  PParamMax=[]  IParamMin=[]  IParamMax=[]  DParamMin=[]  DParamMax=[]  NParamMin=[]  NParamMax=[]  KbParamMin=[]  KbParamMax=[]  KtParamMin=[]  KtParamMax=[]  POutMin=[]  POutMax=[]  IOutMin=[]  IOutMax=[]  DOutMin=[]  DOutMax=[]  NOutMin=[]  NOutMax=[]  KbOutMin=[]  KbOutMax=[]  KtOutMin=[]  KtOutMax=[]  IntegratorOutMin=[]  IntegratorOutMax=[]  FilterOutMin=[]  FilterOutMax=[]  SumOutMin=[]  SumOutMax=[]  SumI1OutMin=[]  SumI1OutMax=[]  SumI2OutMin=[]  SumI2OutMax=[]  SumI3OutMin=[]  SumI3OutMax=[]  SumDOutMin=[]  SumDOutMax=[]  SaturationOutMin=[]  SaturationOutMax=[]  IntegratorContinuousStateAttributes=''  IntegratorStateMustResolveToSignalObject=off  IntegratorRTWStateStorageClass=Auto  FilterContinuousStateAttributes=''  FilterStateMustResolveToSignalObject=off  FilterRTWStateStorageClass=Auto  DifferentiatorICPrevScaledInput=0  DifferentiatorOutMin=[]  DifferentiatorOutMax=[]
  Gain : Gain  Gain=255
  Saturation : Saturate  UpperLimit=1  LowerLimit=0
  Saturation1 : Saturate  UpperLimit=1  LowerLimit=0
  Saturation2 : Saturate  UpperLimit=1  LowerLimit=0
  Sign : Signum
  Unary Minus : UnaryMinus
  PWM : Outport
  INA : Outport  Port=2
  INB : Outport  Port=3
  wires:
  feedback/1 -> Add/2
  Abs/1 -> Saturation2/1
  Sign/1 -> Unary Minus/1, Saturation/1
  Discrete PID Controller/1 -> Abs/1, Sign/1
  Saturation/1 -> INA/1
  Saturation1/1 -> INB/1
  Unary Minus/1 -> Saturation1/1
  target/1 -> Add/1
  Saturation2/1 -> Gain/1
  Gain/1 -> PWM/1
  Add/1 -> Discrete PID Controller/1

== system TITAN_20160720_lec/FrSystem 3/Motor Ctrl FR3 ==
  target : Inport
  feedback : Inport  Port=2
  Abs : Abs
  Add : Sum  Inputs=+-
  Discrete PID Controller : simulink/Continuous/PID Controller  Controller=PID  TimeDomain=Discrete-time  SampleTime=SampleTime  IntegratorMethod=Trapezoidal  FilterMethod=Forward Euler  Form=Parallel  UseFilter=on  ControllerParametersSource=internal  P=0.3  I=0  D=0  N=100  InitialConditionSource=internal  InitialConditionForIntegrator=0  InitialConditionForFilter=0  ExternalReset=none  LimitOutput=on  UpperSaturationLimit=1  LowerSaturationLimit=-1  LinearizeAsGain=off  AntiWindupMode=none  Kb=1  TrackingMode=off  Kt=1  PParamMin=[]  PParamMax=[]  IParamMin=[]  IParamMax=[]  DParamMin=[]  DParamMax=[]  NParamMin=[]  NParamMax=[]  KbParamMin=[]  KbParamMax=[]  KtParamMin=[]  KtParamMax=[]  POutMin=[]  POutMax=[]  IOutMin=[]  IOutMax=[]  DOutMin=[]  DOutMax=[]  NOutMin=[]  NOutMax=[]  KbOutMin=[]  KbOutMax=[]  KtOutMin=[]  KtOutMax=[]  IntegratorOutMin=[]  IntegratorOutMax=[]  FilterOutMin=[]  FilterOutMax=[]  SumOutMin=[]  SumOutMax=[]  SumI1OutMin=[]  SumI1OutMax=[]  SumI2OutMin=[]  SumI2OutMax=[]  SumI3OutMin=[]  SumI3OutMax=[]  SumDOutMin=[]  SumDOutMax=[]  SaturationOutMin=[]  SaturationOutMax=[]  IntegratorContinuousStateAttributes=''  IntegratorStateMustResolveToSignalObject=off  IntegratorRTWStateStorageClass=Auto  FilterContinuousStateAttributes=''  FilterStateMustResolveToSignalObject=off  FilterRTWStateStorageClass=Auto  DifferentiatorICPrevScaledInput=0  DifferentiatorOutMin=[]  DifferentiatorOutMax=[]
  Gain : Gain  Gain=255
  Saturation : Saturate  UpperLimit=1  LowerLimit=0
  Saturation1 : Saturate  UpperLimit=1  LowerLimit=0
  Saturation2 : Saturate  LowerLimit=0
  Sign : Signum
  Unary Minus : UnaryMinus
  PWM : Outport
  INA : Outport  Port=2
  INB : Outport  Port=3
  wires:
  feedback/1 -> Add/2
  Abs/1 -> Saturation2/1
  Sign/1 -> Unary Minus/1, Saturation/1
  Discrete PID Controller/1 -> Abs/1, Sign/1
  Saturation/1 -> INA/1
  Saturation1/1 -> INB/1
  Unary Minus/1 -> Saturation1/1
  target/1 -> Add/1
  Saturation2/1 -> Gain/1
  Gain/1 -> PWM/1
  Add/1 -> Discrete PID Controller/1

== system TITAN_20160720_lec/RlSystem 1/Motor Ctrl FL4 ==
  target : Inport
  feedback : Inport  Port=2
  Abs : Abs
  Add : Sum  Inputs=+-
  Discrete PID Controller : simulink/Continuous/PID Controller  Controller=PID  TimeDomain=Discrete-time  SampleTime=SampleTime  IntegratorMethod=Trapezoidal  FilterMethod=Forward Euler  Form=Parallel  UseFilter=on  ControllerParametersSource=internal  P=0.25  I=0  D=0  N=100  InitialConditionSource=internal  InitialConditionForIntegrator=0  InitialConditionForFilter=0  ExternalReset=none  LimitOutput=on  UpperSaturationLimit=1  LowerSaturationLimit=-1  LinearizeAsGain=off  AntiWindupMode=none  Kb=1  TrackingMode=off  Kt=1  PParamMin=[]  PParamMax=[]  IParamMin=[]  IParamMax=[]  DParamMin=[]  DParamMax=[]  NParamMin=[]  NParamMax=[]  KbParamMin=[]  KbParamMax=[]  KtParamMin=[]  KtParamMax=[]  POutMin=[]  POutMax=[]  IOutMin=[]  IOutMax=[]  DOutMin=[]  DOutMax=[]  NOutMin=[]  NOutMax=[]  KbOutMin=[]  KbOutMax=[]  KtOutMin=[]  KtOutMax=[]  IntegratorOutMin=[]  IntegratorOutMax=[]  FilterOutMin=[]  FilterOutMax=[]  SumOutMin=[]  SumOutMax=[]  SumI1OutMin=[]  SumI1OutMax=[]  SumI2OutMin=[]  SumI2OutMax=[]  SumI3OutMin=[]  SumI3OutMax=[]  SumDOutMin=[]  SumDOutMax=[]  SaturationOutMin=[]  SaturationOutMax=[]  IntegratorContinuousStateAttributes=''  IntegratorStateMustResolveToSignalObject=off  IntegratorRTWStateStorageClass=Auto  FilterContinuousStateAttributes=''  FilterStateMustResolveToSignalObject=off  FilterRTWStateStorageClass=Auto  DifferentiatorICPrevScaledInput=0  DifferentiatorOutMin=[]  DifferentiatorOutMax=[]
  Gain : Gain  Gain=255
  Saturation : Saturate  UpperLimit=1  LowerLimit=0
  Saturation1 : Saturate  UpperLimit=1  LowerLimit=0
  Saturation2 : Saturate  UpperLimit=1  LowerLimit=0
  Sign : Signum
  Unary Minus : UnaryMinus
  PWM : Outport
  INA : Outport  Port=2
  INB : Outport  Port=3
  wires:
  feedback/1 -> Add/2
  Abs/1 -> Saturation2/1
  Sign/1 -> Unary Minus/1, Saturation/1
  Discrete PID Controller/1 -> Abs/1, Sign/1
  Saturation/1 -> INA/1
  Saturation1/1 -> INB/1
  Unary Minus/1 -> Saturation1/1
  target/1 -> Add/1
  Saturation2/1 -> Gain/1
  Gain/1 -> PWM/1
  Add/1 -> Discrete PID Controller/1

== system TITAN_20160720_lec/RlSystem 2/Motor Ctrl FL5 ==
  target : Inport
  feedback : Inport  Port=2
  Abs : Abs
  Add : Sum  Inputs=+-
  Discrete PID Controller : simulink/Continuous/PID Controller  Controller=PID  TimeDomain=Discrete-time  SampleTime=SampleTime  IntegratorMethod=Trapezoidal  FilterMethod=Forward Euler  Form=Parallel  UseFilter=on  ControllerParametersSource=internal  P=0.5  I=0  D=0  N=100  InitialConditionSource=internal  InitialConditionForIntegrator=0  InitialConditionForFilter=0  ExternalReset=none  LimitOutput=on  UpperSaturationLimit=1  LowerSaturationLimit=-1  LinearizeAsGain=off  AntiWindupMode=none  Kb=1  TrackingMode=off  Kt=1  PParamMin=[]  PParamMax=[]  IParamMin=[]  IParamMax=[]  DParamMin=[]  DParamMax=[]  NParamMin=[]  NParamMax=[]  KbParamMin=[]  KbParamMax=[]  KtParamMin=[]  KtParamMax=[]  POutMin=[]  POutMax=[]  IOutMin=[]  IOutMax=[]  DOutMin=[]  DOutMax=[]  NOutMin=[]  NOutMax=[]  KbOutMin=[]  KbOutMax=[]  KtOutMin=[]  KtOutMax=[]  IntegratorOutMin=[]  IntegratorOutMax=[]  FilterOutMin=[]  FilterOutMax=[]  SumOutMin=[]  SumOutMax=[]  SumI1OutMin=[]  SumI1OutMax=[]  SumI2OutMin=[]  SumI2OutMax=[]  SumI3OutMin=[]  SumI3OutMax=[]  SumDOutMin=[]  SumDOutMax=[]  SaturationOutMin=[]  SaturationOutMax=[]  IntegratorContinuousStateAttributes=''  IntegratorStateMustResolveToSignalObject=off  IntegratorRTWStateStorageClass=Auto  FilterContinuousStateAttributes=''  FilterStateMustResolveToSignalObject=off  FilterRTWStateStorageClass=Auto  DifferentiatorICPrevScaledInput=0  DifferentiatorOutMin=[]  DifferentiatorOutMax=[]
  Gain : Gain  Gain=255
  Saturation : Saturate  UpperLimit=1  LowerLimit=0
  Saturation1 : Saturate  UpperLimit=1  LowerLimit=0
  Saturation2 : Saturate  UpperLimit=1  LowerLimit=0
  Sign : Signum
  Unary Minus : UnaryMinus
  PWM : Outport
  INA : Outport  Port=2
  INB : Outport  Port=3
  wires:
  feedback/1 -> Add/2
  Abs/1 -> Saturation2/1
  Sign/1 -> Unary Minus/1, Saturation/1
  Discrete PID Controller/1 -> Abs/1, Sign/1
  Saturation/1 -> INA/1
  Saturation1/1 -> INB/1
  Unary Minus/1 -> Saturation1/1
  target/1 -> Add/1
  Saturation2/1 -> Gain/1
  Gain/1 -> PWM/1
  Add/1 -> Discrete PID Controller/1

== system TITAN_20160720_lec/RlSystem 3/Motor Ctrl FL6 ==
  target : Inport
  feedback : Inport  Port=2
  Abs : Abs
  Add : Sum  Inputs=+-
  Discrete PID Controller : simulink/Continuous/PID Controller  Controller=PID  TimeDomain=Discrete-time  SampleTime=SampleTime  IntegratorMethod=Trapezoidal  FilterMethod=Forward Euler  Form=Parallel  UseFilter=on  ControllerParametersSource=internal  P=0.35  I=0  D=0  N=100  InitialConditionSource=internal  InitialConditionForIntegrator=0  InitialConditionForFilter=0  ExternalReset=none  LimitOutput=on  UpperSaturationLimit=1  LowerSaturationLimit=-1  LinearizeAsGain=off  AntiWindupMode=none  Kb=1  TrackingMode=off  Kt=1  PParamMin=[]  PParamMax=[]  IParamMin=[]  IParamMax=[]  DParamMin=[]  DParamMax=[]  NParamMin=[]  NParamMax=[]  KbParamMin=[]  KbParamMax=[]  KtParamMin=[]  KtParamMax=[]  POutMin=[]  POutMax=[]  IOutMin=[]  IOutMax=[]  DOutMin=[]  DOutMax=[]  NOutMin=[]  NOutMax=[]  KbOutMin=[]  KbOutMax=[]  KtOutMin=[]  KtOutMax=[]  IntegratorOutMin=[]  IntegratorOutMax=[]  FilterOutMin=[]  FilterOutMax=[]  SumOutMin=[]  SumOutMax=[]  SumI1OutMin=[]  SumI1OutMax=[]  SumI2OutMin=[]  SumI2OutMax=[]  SumI3OutMin=[]  SumI3OutMax=[]  SumDOutMin=[]  SumDOutMax=[]  SaturationOutMin=[]  SaturationOutMax=[]  IntegratorContinuousStateAttributes=''  IntegratorStateMustResolveToSignalObject=off  IntegratorRTWStateStorageClass=Auto  FilterContinuousStateAttributes=''  FilterStateMustResolveToSignalObject=off  FilterRTWStateStorageClass=Auto  DifferentiatorICPrevScaledInput=0  DifferentiatorOutMin=[]  DifferentiatorOutMax=[]
  Gain : Gain  Gain=255
  Saturation : Saturate  UpperLimit=1  LowerLimit=0
  Saturation1 : Saturate  UpperLimit=1  LowerLimit=0
  Saturation2 : Saturate  LowerLimit=0
  Sign : Signum
  Unary Minus : UnaryMinus
  PWM : Outport
  INA : Outport  Port=2
  INB : Outport  Port=3
  wires:
  feedback/1 -> Add/2
  Abs/1 -> Saturation2/1
  Sign/1 -> Unary Minus/1, Saturation/1
  Discrete PID Controller/1 -> Abs/1, Sign/1
  Saturation/1 -> INA/1
  Saturation1/1 -> INB/1
  Unary Minus/1 -> Saturation1/1
  target/1 -> Add/1
  Saturation2/1 -> Gain/1
  Gain/1 -> PWM/1
  Add/1 -> Discrete PID Controller/1

== system TITAN_20160720_lec/RrSystem 1/Motor Ctrl RR1 ==
  target : Inport
  feedback : Inport  Port=2
  Abs : Abs
  Add : Sum  Inputs=+-
  Discrete PID Controller : simulink/Continuous/PID Controller  Controller=PID  TimeDomain=Discrete-time  SampleTime=SampleTime  IntegratorMethod=Trapezoidal  FilterMethod=Forward Euler  Form=Parallel  UseFilter=on  ControllerParametersSource=internal  P=0.5  I=0  D=0  N=100  InitialConditionSource=internal  InitialConditionForIntegrator=0  InitialConditionForFilter=0  ExternalReset=none  LimitOutput=on  UpperSaturationLimit=1  LowerSaturationLimit=-1  LinearizeAsGain=off  AntiWindupMode=none  Kb=1  TrackingMode=off  Kt=1  PParamMin=[]  PParamMax=[]  IParamMin=[]  IParamMax=[]  DParamMin=[]  DParamMax=[]  NParamMin=[]  NParamMax=[]  KbParamMin=[]  KbParamMax=[]  KtParamMin=[]  KtParamMax=[]  POutMin=[]  POutMax=[]  IOutMin=[]  IOutMax=[]  DOutMin=[]  DOutMax=[]  NOutMin=[]  NOutMax=[]  KbOutMin=[]  KbOutMax=[]  KtOutMin=[]  KtOutMax=[]  IntegratorOutMin=[]  IntegratorOutMax=[]  FilterOutMin=[]  FilterOutMax=[]  SumOutMin=[]  SumOutMax=[]  SumI1OutMin=[]  SumI1OutMax=[]  SumI2OutMin=[]  SumI2OutMax=[]  SumI3OutMin=[]  SumI3OutMax=[]  SumDOutMin=[]  SumDOutMax=[]  SaturationOutMin=[]  SaturationOutMax=[]  IntegratorContinuousStateAttributes=''  IntegratorStateMustResolveToSignalObject=off  IntegratorRTWStateStorageClass=Auto  FilterContinuousStateAttributes=''  FilterStateMustResolveToSignalObject=off  FilterRTWStateStorageClass=Auto  DifferentiatorICPrevScaledInput=0  DifferentiatorOutMin=[]  DifferentiatorOutMax=[]
  Gain : Gain  Gain=255
  Saturation : Saturate  UpperLimit=1  LowerLimit=0
  Saturation1 : Saturate  UpperLimit=1  LowerLimit=0
  Saturation2 : Saturate  UpperLimit=1  LowerLimit=0
  Sign : Signum
  Unary Minus : UnaryMinus
  PWM : Outport
  INA : Outport  Port=2
  INB : Outport  Port=3
  wires:
  feedback/1 -> Add/2
  Abs/1 -> Saturation2/1
  Sign/1 -> Unary Minus/1, Saturation/1
  Discrete PID Controller/1 -> Abs/1, Sign/1
  Saturation/1 -> INA/1
  Saturation1/1 -> INB/1
  Unary Minus/1 -> Saturation1/1
  target/1 -> Add/1
  Saturation2/1 -> Gain/1
  Gain/1 -> PWM/1
  Add/1 -> Discrete PID Controller/1

== system TITAN_20160720_lec/RrSystem 2/Motor Ctrl RR2 ==
  target : Inport
  feedback : Inport  Port=2
  Abs : Abs
  Add : Sum  Inputs=+-
  Discrete PID Controller : simulink/Continuous/PID Controller  Controller=PID  TimeDomain=Discrete-time  SampleTime=SampleTime  IntegratorMethod=Trapezoidal  FilterMethod=Forward Euler  Form=Parallel  UseFilter=on  ControllerParametersSource=internal  P=0.3  I=0  D=0  N=100  InitialConditionSource=internal  InitialConditionForIntegrator=0  InitialConditionForFilter=0  ExternalReset=none  LimitOutput=on  UpperSaturationLimit=1  LowerSaturationLimit=-1  LinearizeAsGain=off  AntiWindupMode=none  Kb=1  TrackingMode=off  Kt=1  PParamMin=[]  PParamMax=[]  IParamMin=[]  IParamMax=[]  DParamMin=[]  DParamMax=[]  NParamMin=[]  NParamMax=[]  KbParamMin=[]  KbParamMax=[]  KtParamMin=[]  KtParamMax=[]  POutMin=[]  POutMax=[]  IOutMin=[]  IOutMax=[]  DOutMin=[]  DOutMax=[]  NOutMin=[]  NOutMax=[]  KbOutMin=[]  KbOutMax=[]  KtOutMin=[]  KtOutMax=[]  IntegratorOutMin=[]  IntegratorOutMax=[]  FilterOutMin=[]  FilterOutMax=[]  SumOutMin=[]  SumOutMax=[]  SumI1OutMin=[]  SumI1OutMax=[]  SumI2OutMin=[]  SumI2OutMax=[]  SumI3OutMin=[]  SumI3OutMax=[]  SumDOutMin=[]  SumDOutMax=[]  SaturationOutMin=[]  SaturationOutMax=[]  IntegratorContinuousStateAttributes=''  IntegratorStateMustResolveToSignalObject=off  IntegratorRTWStateStorageClass=Auto  FilterContinuousStateAttributes=''  FilterStateMustResolveToSignalObject=off  FilterRTWStateStorageClass=Auto  DifferentiatorICPrevScaledInput=0  DifferentiatorOutMin=[]  DifferentiatorOutMax=[]
  Gain : Gain  Gain=255
  Saturation : Saturate  UpperLimit=1  LowerLimit=0
  Saturation1 : Saturate  UpperLimit=1  LowerLimit=0
  Saturation2 : Saturate  UpperLimit=1  LowerLimit=0
  Sign : Signum
  Unary Minus : UnaryMinus
  PWM : Outport
  INA : Outport  Port=2
  INB : Outport  Port=3
  wires:
  feedback/1 -> Add/2
  Abs/1 -> Saturation2/1
  Sign/1 -> Unary Minus/1, Saturation/1
  Discrete PID Controller/1 -> Abs/1, Sign/1
  Saturation/1 -> INA/1
  Saturation1/1 -> INB/1
  Unary Minus/1 -> Saturation1/1
  target/1 -> Add/1
  Saturation2/1 -> Gain/1
  Gain/1 -> PWM/1
  Add/1 -> Discrete PID Controller/1

== system TITAN_20160720_lec/RrSystem 3/Motor Ctrl RR3 ==
  target : Inport
  feedback : Inport  Port=2
  Abs : Abs
  Add : Sum  Inputs=+-
  Discrete PID Controller : simulink/Continuous/PID Controller  Controller=PID  TimeDomain=Discrete-time  SampleTime=SampleTime  IntegratorMethod=Trapezoidal  FilterMethod=Forward Euler  Form=Parallel  UseFilter=on  ControllerParametersSource=internal  P=0.3  I=0  D=0  N=100  InitialConditionSource=internal  InitialConditionForIntegrator=0  InitialConditionForFilter=0  ExternalReset=none  LimitOutput=on  UpperSaturationLimit=1  LowerSaturationLimit=-1  LinearizeAsGain=off  AntiWindupMode=none  Kb=1  TrackingMode=off  Kt=1  PParamMin=[]  PParamMax=[]  IParamMin=[]  IParamMax=[]  DParamMin=[]  DParamMax=[]  NParamMin=[]  NParamMax=[]  KbParamMin=[]  KbParamMax=[]  KtParamMin=[]  KtParamMax=[]  POutMin=[]  POutMax=[]  IOutMin=[]  IOutMax=[]  DOutMin=[]  DOutMax=[]  NOutMin=[]  NOutMax=[]  KbOutMin=[]  KbOutMax=[]  KtOutMin=[]  KtOutMax=[]  IntegratorOutMin=[]  IntegratorOutMax=[]  FilterOutMin=[]  FilterOutMax=[]  SumOutMin=[]  SumOutMax=[]  SumI1OutMin=[]  SumI1OutMax=[]  SumI2OutMin=[]  SumI2OutMax=[]  SumI3OutMin=[]  SumI3OutMax=[]  SumDOutMin=[]  SumDOutMax=[]  SaturationOutMin=[]  SaturationOutMax=[]  IntegratorContinuousStateAttributes=''  IntegratorStateMustResolveToSignalObject=off  IntegratorRTWStateStorageClass=Auto  FilterContinuousStateAttributes=''  FilterStateMustResolveToSignalObject=off  FilterRTWStateStorageClass=Auto  DifferentiatorICPrevScaledInput=0  DifferentiatorOutMin=[]  DifferentiatorOutMax=[]
  Gain : Gain  Gain=255
  Saturation : Saturate  UpperLimit=1  LowerLimit=0
  Saturation1 : Saturate  UpperLimit=1  LowerLimit=0
  Saturation2 : Saturate  LowerLimit=0
  Sign : Signum
  Unary Minus : UnaryMinus
  PWM : Outport
  INA : Outport  Port=2
  INB : Outport  Port=3
  wires:
  feedback/1 -> Add/2
  Abs/1 -> Saturation2/1
  Sign/1 -> Unary Minus/1, Saturation/1
  Discrete PID Controller/1 -> Abs/1, Sign/1
  Saturation/1 -> INA/1
  Saturation1/1 -> INB/1
  Unary Minus/1 -> Saturation1/1
  target/1 -> Add/1
  Saturation2/1 -> Gain/1
  Gain/1 -> PWM/1
  Add/1 -> Discrete PID Controller/1
